simulink model "Connecting_to_ROS_Robot_2"  (R2017b)
settings: Solver=VariableStepAuto  StartTime=0.0  StopTime=inf  RelTol=1e-3
undefined symbols (not defined in the file): Angular, Linear
libraries: robotlib x3, simulink x3
settings Model: Creator=root  LastModifiedBy=root

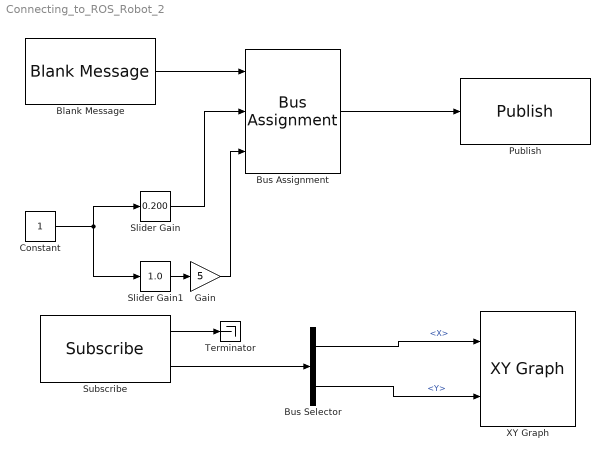
== system Connecting_to_ROS_Robot_2 ==
  Blank Message : robotlib/Blank Message  SourceLibraryInfo=This block requires Robotics System Toolbox  messageType=geometry_msgs/Twist  SampleTime=.01
      settings: SourceProductBaseCode=RO
  Bus Assignment : BusAssignment  AssignedSignals=Linear.X,Angular.Z
  Bus Selector : BusSelector  OutputSignals=Pose.Pose.Position.X,Pose.Pose.Position.Y
  Constant : Constant
  Gain : Gain  Gain=5
  Publish : robotlib/Publish  SourceLibraryInfo=This block requires Robotics System Toolbox  topicSource=Select from ROS network  topic=/mobile_base/commands/velocity  messageType=geometry_msgs/Twist  messageQueueLength=1
      settings: SourceProductBaseCode=RO
  Slider Gain : simulink/Math Operations/Slider Gain  gain=0.200  low=0  high=2
  Slider Gain1 : simulink/Math Operations/Slider Gain  gain=1.0  low=-1  high=1
  Subscribe : robotlib/Subscribe  SourceLibraryInfo=This block requires Robotics System Toolbox  topicSource=Select from ROS network  topic=/odom  messageType=nav_msgs/Odometry  sampleTime=-1  messageQueueLength=1
      settings: SourceProductBaseCode=RO
  Terminator : Terminator
  XY Graph : simulink/Sinks/XY Graph  xmin=-1  xmax=1  ymin=-1  ymax=1  st=-1
  wires:
  Slider Gain1/1 -> Gain/1
  Slider Gain/1 -> Bus Assignment/2
  Constant/1 -> Slider Gain1/1, Slider Gain/1
  Subscribe/1 -> Terminator/1
  Bus Selector/1 -> XY Graph/1  "<X>"
  Bus Selector/2 -> XY Graph/2  "<Y>"
  Gain/1 -> Bus Assignment/3
  Blank Message/1 -> Bus Assignment/1
  Bus Assignment/1 -> Publish/1
  Subscribe/2 -> Bus Selector/1
